simulink model "merge_1"  (Simulink 4.00)
settings: Solver=ode45  StartTime=0.0  StopTime=10.0  MaxStep=0.01  RelTol=1e-3
libraries: simulink3 x2
settings Model: LastModifiedBy=Administrator  Refine=5  BlockReductionOpt=off

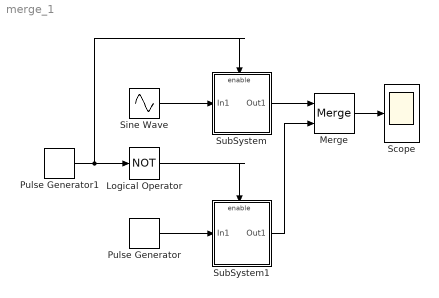
== system merge_1 ==
  Logical Operator : Logic  Operator=NOT  Inputs=2
  Merge : Merge  Inputs=2  InitialOutput=[1]  AllowUnequalInputPortWidths=off  InputPortOffsets=[]
  Pulse Generator : simulink3/Sources/Pulse Generator  period=0.2  duty=50  amplitude=1  start=0
  Pulse Generator1 : simulink3/Sources/Pulse Generator  period=2  duty=50  amplitude=1  start=0
  Scope : Scope
      settings: TimeRange=5  YMin=-5  YMax=5  SaveToWorkspace=off  SaveName=ScopeData  LimitDataPoints=on  MaxDataPoints=5000
  Sine Wave : Sin  Amplitude=1  Frequency=2*pi*10  Phase=0  SampleTime=0
  SubSystem : Subsystem  TreatAsAtomicUnit=on
      settings: RTWFcnNameOpts=Auto  RTWFileNameOpts=Auto
  SubSystem1 : Subsystem  TreatAsAtomicUnit=on
      settings: RTWFcnNameOpts=Auto  RTWFileNameOpts=Auto
  wires:
  Merge/1 -> Scope/1
  Sine Wave/1 -> SubSystem/1(In1)
  Pulse Generator/1 -> SubSystem1/1(In1)
  Pulse Generator1/1 -> SubSystem/Enable, Logical Operator/1
  Logical Operator/1 -> SubSystem1/Enable
  SubSystem1/1(Out1) -> Merge/2
  SubSystem/1(Out1) -> Merge/1

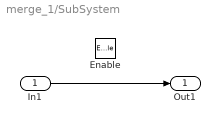
== system merge_1/SubSystem ==
  In1 : Inport  Port=1
  Enable : EnablePort
  Out1 : Outport  Port=1
  wires:
  In1/1 -> Out1/1

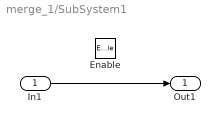
== system merge_1/SubSystem1 ==
  In1 : Inport  Port=1
  Enable : EnablePort
  Out1 : Outport  Port=1
  wires:
  In1/1 -> Out1/1
